simulink model "GFo_29bus"  (R2020a)
settings: Solver=ode1  StartTime=0.0  StopTime=4.5  FixedStep=Time_Step  RelTol=1e-3  EnableMultiTasking=on
PreLoadFcn:
  | Init_29bus;
InitFcn:
  | Init_29bus;
undefined symbols (not defined in the file): D1, D11, Delta, Time_Step, VSC01_Delta_P_Time_Step, VSC01_Delta_P_Value
libraries: powerlib x175, GFo_Lib x1
(part 1 of 5)
Description:
  | Copyright 2008-2017 The MathWorks, Inc.
settings Model: Creator=MathWorks  LastModifiedBy=Frederic_Colas
settings DataIOCC: SaveFormat=StructureWithTime  SignalLoggingSaveFormat=ModelDataLogs  SaveOutput=off  SignalLogging=off  DSMLogging=off  SaveTime=off  ReturnWorkspaceOutputs=off
settings OptimizationCC: ExpressionDepthLimit=2147483647  LifeSpan=inf
settings DebuggingCC: UnderspecifiedInitializationDetection=Classic  MergeDetectMultiDrivingBlocksExec=none  SolverPrmCheckMsg=warning  FcnCallInpInsideContextMsg=warning  UnconnectedInputMsg=none  UnconnectedOutputMsg=none  UnconnectedLineMsg=none  StateNameClashWarn=warning  SFUnexpectedBacktrackingDiag=warning  SFNoUnconditionalDefaultTransitionDiag=warning  SFExecutionAtInitializationDiag=none  ArithmeticOperatorsInVariantConditions=warning
settings HardwareCC: ProdBitPerPointer=32  ProdBitPerSizeT=32  ProdBitPerPtrDiffT=32  ProdLargestAtomicFloat=None  ProdIntDivRoundTo=Undefined  ProdEndianess=Unspecified  ProdWordSize=32  ProdHWDeviceType=32-bit Generic
settings ModelReferenceCC: PropagateSignalLabelsOutOfModel=off
settings SFSimCC: SimUseLocalCustomCode=off  CustomCodeUndefinedFunction=UseInterfaceOnly
settings RTWCC: RTWUseLocalCustomCode=off
settings CodeAppCC: StateflowObjectComments=on
settings GRTTargetCC: TargetLangStandard=C89/C90 (ANSI)  CombineOutputUpdateFcns=off  GRTInterface=on
settings ConfigComp: CovMetricSettings=dw  CovSaveCumulativeToWorkspaceVar=on  CovSaveSingleToWorkspaceVar=on  CovExternalEMLEnable=off  CovSFcnEnable=off
settings SimscapeCC: SimscapeNormalizeSystem=off

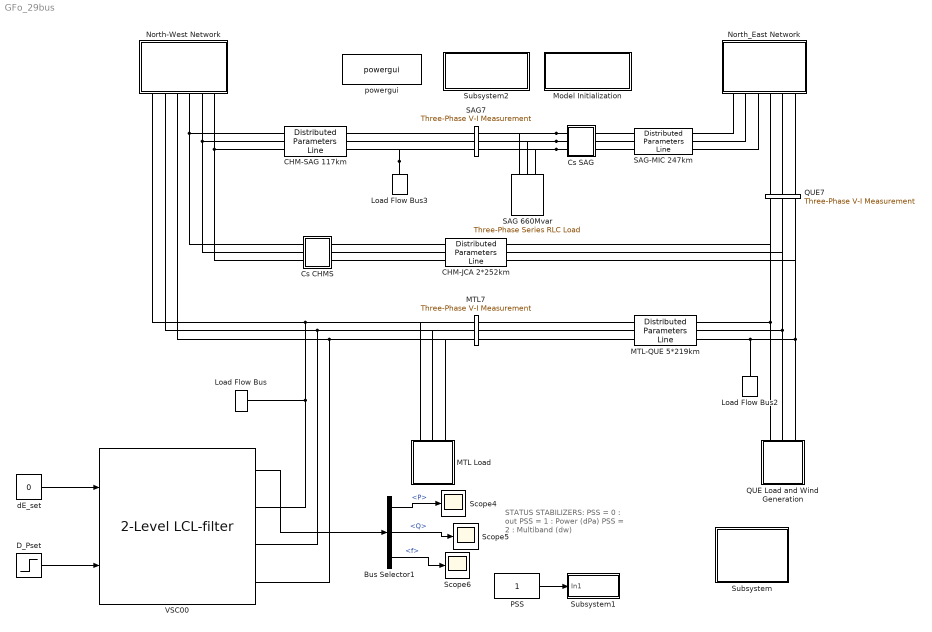
== system GFo_29bus ==
  note: STATUS STABILIZERS:
      | PSS = 0 :  out
      | PSS = 1 :  Power (dPa)
      | PSS = 2 :  Multiband (dw)
  Bus Selector1 : BusSelector  OutputSignals=P,Q,f
  CHM-JCA 2*252km : powerlib/Elements/Distributed Parameters Line  Phases=3  Length=252  Frequency=60  Resistance="[0.01273  0.3864]/2"  Inductance="[0.9337e-3  4.1264e-3]/2"  Capacitance=[12.74e-9 7.751e-9]*2  x1=[-0.00144 1.06587715150696e-07 0 0;-0.0014 1.06951259001269e-07 0 0;-0.00136 1.07290483057854e-07 0 0;-0.00132 1.07605310183825e-07 0 0;-0.00128 1.07895668790209e-07 0 0;-0.00124 1.08161492851963e-07 0 0;-0.0012 1.08402721922987e-07 0 0;-0.00116 1.08619301149872e-07 0 0;-0.00112 1.08811181284367e-07 0 0;-0.00108 1.08978318694587e-07 0 0;-0.00104 1.09120675374924e-07 0 0;-0.001 1.09238218954698e-07 0 0;-0.00096 1.09330922705511e-07 0 0;-0.00092 1.09398765547331e-07 0 0;-0.00088 1.0944173205328e-07 236947.551929989 -735006.025980386;-0.00084 1.09459812453146e-07 248003.849356371 -731349.489712214;-0.0008 1.09453002635601e-07 259003.752846105 -727526.650876972;-0.00076 1.09421304149139e-07 269944.761115994 -723538.378755243;-0.00072 1.09364724201723e-07 280824.38627511 -719385.580245714;-0.00068 1.09283275659145e-07 291640.154390513 -715069.199658954;-0.00064 1.09176977042101e-07 302389.606049806 -710590.218502686;-0.0006 1.09045852521979e-07 313070.296920379 -705949.655258599;-0.00056 1.08889931915365e-07 323679.798305237 -701148.565150758;-0.00052 1.08709250677261e-07 334215.697695255 -696188.039905648;-0.00048 1.08503849893021e-07 344675.599317771 -691069.207503934;-0.00044 1.08273776269012e-07 355057.124681358 -685793.231923961;-0.0004 1.08019082121994e-07 365357.913116674 -680361.312877077;-0.00036 1.07739825367218e-07 375575.62231326 -674774.685534831;-0.00032 1.07436069505262e-07 385707.928852159 -669034.620248103;-0.00028 1.07107883607589e-07 395752.52873424 -663142.42225824;-0.00024 1.06755342300844e-07 405707.137904111 -657099.431400252;-0.0002 1.06378525749878e-07 415569.492769492 -650907.021798148;-0.00016 1.05977519639526e-07 425337.350715936 -644566.60155247;-0.00012 1.05552415155119e-07 435008.49061678 -638079.612420104;-8e-05 1.05103308961751e-07 444580.713338212 -631447.529486439;-4e-05 1.04630303182297e-07 454051.842239331 -624671.860829939]  x2=[-0.00144 7.1019300205437e-08 0 0;-0.0014 7.11442792046729e-08 0 0;-0.00136 7.12530806083399e-08 0 0;-0.00132 7.13456796759369e-08 0 0;-0.00128 7.14220553512345e-08 0 0;-0.00124 7.14821902670629e-08 0 0;-0.0012 7.15260707492606e-08 0 0;-0.00116 7.15536868197846e-08 0 0;-0.00112 7.15650321989784e-08 0 0;-0.00108 7.15601043070008e-08 0 0;-0.00104 7.15389042644118e-08 0 0;-0.001 7.15014368919183e-08 0 0;-0.00096 7.14477107092777e-08 0 0;-0.00092 7.13777379333606e-08 0 0;-0.00088 7.12915344753729e-08 28167.854478783 -750122.429836815;-0.00084 7.11891199372375e-08 39475.8227938335 -749612.37045183;-0.0008 7.10705176071372e-08 50774.8146472057 -748931.855678186;-0.00076 7.09357544542191e-08 62062.2607455905 -748081.040259074;-0.00072 7.0784861122462e-08 73335.5944210838 -747060.117662583;-0.00068 7.06178719237082e-08 84592.2522148251 -745869.320037708;-0.00064 7.04348248298616e-08 95829.6744599052 -744508.91816156;-0.0006 7.02357614642528e-08 107045.305863413 -742979.221377793;-0.00056 7.00207270921744e-08 118236.596087487 -741280.577526264;-0.00052 6.97897706105883e-08 129401.00032924 -739413.372863938;-0.00048 6.95429445370066e-08 140535.979899424 -737378.031977051;-0.00044 6.92803049975501e-08 151639.00279971 -735175.017684571;-0.0004 6.90019117141851e-08 162707.544298438 -732804.830932948;-0.00036 6.87078279911433e-08 173739.087504723 -730268.010682211;-0.00032 6.83981207005275e-08 184731.123940772 -727565.133783408;-0.00028 6.80728602671046e-08 195681.15411229 -724696.814847437;-0.00024 6.77321206522923e-08 206586.688076845 -721663.706105289;-0.0002 6.73759793373407e-08 217445.246010059 -718466.497259735;-0.00016 6.70045173057134e-08 228254.358769498 -715105.915328495;-0.00012 6.66178190246732e-08 239011.568456135 -711582.724478921;-8e-05 6.62159724260743e-08 249714.428973253 -707897.725854228;-4e-05 6.5799068886368e-08 260360.506582668 -704051.757391326]  x3=[-0.00144 2.8189905940601e-10 0 0;-0.0014 2.81135422203296e-10 0 0;-0.00136 2.80307857229982e-10 0 0;-0.00132 2.79416552667206e-10 0 0;-0.00128 2.78461711189939e-10 0 0;-0.00124 2.77443549920899e-10 0 0;-0.0012 2.76362300381179e-10 0 0;-0.00116 2.75218208437598e-10 0 0;-0.00112 2.740115342468e-10 0 0;-0.00108 2.72742552196089e-10 0 0;-0.00104 2.7141155084104e-10 0 0;-0.001 2.70018832839883e-10 0 0;-0.00096 2.68564714884681e-10 0 0;-0.00092 2.67049527629319e-10 0 0;-0.00088 2.6547361561431e-10 329.831041711369 -923.135468483982;-0.00084 2.63837337188458e-10 343.713540361162 -918.056958478673;-0.0008 2.62141064427365e-10 357.517881515936 -912.769690237991;-0.00076 2.6038518304883e-10 371.240926187556 -907.27486604114;-0.00072 2.58570092325136e-10 384.879553874007 -901.573735363756;-0.00068 2.56696204992261e-10 398.430663268966 -895.667594593792;-0.00064 2.54763947156024e-10 411.891172967018 -889.557786736725;-0.0006 2.52773758195194e-10 425.258022164335 -883.245701110174;-0.00056 2.50726090661579e-10 438.528171354681 -876.732773027977;-0.00052 2.48621410177118e-10 451.698603020568 -870.020483473815;-0.00048 2.46460195328001e-10 464.766322319409 -863.110358764447;-0.00044 2.4424293755585e-10 477.72835776453 -856.003970202644;-0.0004 2.41970141045959e-10 490.581761900849 -848.702933719881;-0.00036 2.39642322612656e-10 503.323611975108 -841.208909508892;-0.00032 2.37260011581779e-10 515.951010600483 -833.523601646157;-0.00028 2.34823749670311e-10 528.461086415419 -825.648757704409;-0.00024 2.32334090863202e-10 540.850994736558 -817.586168355251;-0.0002 2.29791601287394e-10 553.117918205594 -809.337666961972;-0.00016 2.27196859083092e-10 565.259067429917 -800.905129162656;-0.00012 2.24550454272297e-10 577.271681616892 -792.290472443681;-8e-05 2.21852988624641e-10 589.153029201647 -783.495655703694;-4e-05 2.1910507552055e-10 600.9004084682 -774.522678808179]  x4=[-0.00144 1.33638805948334e-10 0 0;-0.0014 1.37510109756271e-10 0 0;-0.00136 1.41350144951085e-10 0 0;-0.00132 1.4515803834189e-10 0 0;-0.00128 1.48932924046565e-10 0 0;-0.00124 1.52673943688654e-10 0 0;-0.0012 1.56380246592553e-10 0 0;-0.00116 1.60050989976943e-10 0 0;-0.00112 1.63685339146433e-10 0 0;-0.00108 1.67282467681363e-10 0 0;-0.00104 1.70841557625725e-10 0 0;-0.001 1.74361799673157e-10 0 0;-0.00096 1.77842393350976e-10 0 0;-0.00092 1.81282547202195e-10 0 0;-0.00088 1.84681478965494e-10 -191.737879033871 -10272.5482528801;-0.00084 1.88038415753101e-10 -36.8152546198599 -10274.271133571;-0.0008 1.91352594226541e-10 118.11574126557 -10273.6577336076;-0.00076 1.94623260770207e-10 273.019878650024 -10270.7081924719;-0.00072 1.97849671662735e-10 427.861933668495 -10265.423180864;-0.00068 2.01031093246108e-10 582.606696572975 -10257.80390055;-0.00064 2.04166802092497e-10 737.218979738841 -10247.8520840885;-0.0006 2.07256085168748e-10 891.663625666219 -10235.5699944369;-0.00056 2.10298239998533e-10 1045.9055149745 -10220.9604244363;-0.00052 2.13292574822077e-10 1199.90957438818 -10204.026696177;-0.00048 2.16238408753463e-10 1353.64078471223 -10184.7726602428;-0.00044 2.19135071935459e-10 1507.06418879513 -10163.2026948353;-0.0004 2.21981905691838e-10 1660.14489947787 -10139.3217047788;-0.00036 2.24778262677152e-10 1812.84810752694 -10113.1351204044;-0.00032 2.27523507023939e-10 1965.1390895497 -10084.6488963156;-0.00028 2.30217014487308e-10 2116.98321589014 -10053.8695100341;-0.00024 2.3285817258689e-10 2268.34595850337 -10020.8039605269;-0.0002 2.35446380746108e-10 2419.19289880701 -9985.45976661477;-0.00016 2.37981050428748e-10 2569.4897355077 -9947.84496526266;-0.00012 2.40461605272782e-10 2719.20229240087 -9907.96810975201;-8e-05 2.42887481221429e-10 2868.29652614215 -9865.83826773589;-4e-05 2.45258126651419e-10 3016.73853398852 -9821.46501917704]  x5=0.00142516474882927  V1=ones(3,3)  V2=ones(3,3)  I1=ones(3,3)  I2=ones(3,3)  nHarmo=1  Measurements=None  Decoupling=off  VsMag0=0  VrMag0=0  VsAngle0=0  VrAngle0=0  IsMag0=0  IrMag0=0  IsAngle0=0  IrAngle0=0
      settings: AttributesFormatString=\n
  CHM-SAG 117km : powerlib/Elements/Distributed Parameters Line  Phases=3  Length=117  Frequency=60  Resistance="[0.01273  0.3864]"  Inductance="[0.9337e-3  4.1264e-3]"  Capacitance=[12.74e-9 7.751e-9]  x1=[-0.00068 1.07436413044344e-07 0 0;-0.00064 1.07336181458683e-07 0 0;-0.0006 1.07211542550985e-07 0 0;-0.00056 1.07062524663065e-07 0 0;-0.00052 1.06889161680303e-07 0 0;-0.00048 1.06691493023949e-07 0 0;-0.00044 1.06469563642149e-07 285915.250875085 -721016.735544479;-0.0004 1.06223423999732e-07 296755.036612825 -716623.402961044;-0.00036 1.05953130066728e-07 307527.342814346 -712067.116395673;-0.00032 1.05658743305649e-07 318229.719950114 -707348.911908639;-0.00028 1.05340330657504e-07 328859.734391862 -702469.862378953;-0.00024 1.04997964526583e-07 339414.968965975 -697431.077260406;-0.0002 1.04631722763993e-07 349893.023503134 -692233.702329278;-0.00016 1.04241688649953e-07 360291.515384098 -686878.91942381;-0.00012 1.03827950874855e-07 370608.080081486 -681367.946175457;-8e-05 1.03390603519102e-07 380840.371697451 -675702.03573201;-4e-05 1.02929746031712e-07 390986.063497119 -669882.476472644]  x2=[-0.00068 7.37125407254179e-08 0 0;-0.00064 7.3600352625818e-08 0 0;-0.0006 7.34714284407333e-08 0 0;-0.00056 7.33257974864118e-08 0 0;-0.00052 7.31634928780767e-08 0 0;-0.00048 7.29845515223962e-08 0 0;-0.00044 7.27890141090914e-08 332776.301409299 -689011.544372579;-0.0004 7.2576925101684e-08 343128.151600145 -683915.224594401;-0.00036 7.23483327273852e-08 353401.977408328 -678663.388391983;-0.00032 7.21032889661296e-08 363595.442654457 -673257.22998759;-0.00028 7.18418495387554e-08 373706.22943244 -667697.978695019;-0.00024 7.15640738943339e-08 383732.038636556 -661986.898640076;-0.0002 7.1270025196651e-08 393670.590484249 -656125.288473114;-0.00016 7.0959770309845e-08 403519.625034538 -650114.481073737;-0.00012 7.06333797832015e-08 413276.902701898 -643955.843247712;-8e-05 7.02909278351116e-08 422940.204765532 -637650.775416171;-4e-05 6.99324923361951e-08 432507.333873884 -631200.711297167]  x3=[-0.00068 1.02796560750471e-10 0 0;-0.00064 1.00332195956181e-10 0 0;-0.0006 9.7845016485759e-11 0 0;-0.00056 9.53355879023672e-11 0 0;-0.00052 9.28044808284255e-11 0 0;-0.00048 9.02522708158551e-11 0 0;-0.00044 8.76795382152037e-11 1667.28750300207 -3842.30394709124;-0.0004 8.50868680436783e-11 1725.03630670002 -3816.72583715204;-0.00036 8.24748498521176e-11 1782.3928520179 -3790.27983667152;-0.00032 7.98440775909334e-11 1839.34409657194 -3762.97195924212;-0.00028 7.7195149475051e-11 1895.87709014024 -3734.80841443967;-0.00024 7.45286678478806e-11 1951.9789776076 -3705.7956064114;-0.0002 7.18452390443494e-11 2007.6370018886 -3675.94013241965;-0.00016 6.91454732530265e-11 2062.83850682849 -3645.24878134175;-0.00012 6.64299843773711e-11 2117.57094008109 -3613.72853212625;-8e-05 6.3699389896136e-11 2171.82185596306 -3581.38655220602;-4e-05 6.09543107229587e-11 2225.57891828399 -3548.23019586838]  x4=[-0.00068 1.34957667935224e-10 0 0;-0.00064 1.37600660085736e-10 0 0;-0.0006 1.40212363032762e-10 0 0;-0.00056 1.42792182897574e-10 0 0;-0.00052 1.45339533051383e-10 0 0;-0.00048 1.47853834248731e-10 0 0;-0.00044 1.50334514759208e-10 212.800113433279 -1518.35731016245;-0.0004 1.52781010497458e-10 235.671559776652 -1514.97578249147;-0.00036 1.55192765151448e-10 258.489416439676 -1511.24976239214;-0.00032 1.57569230308969e-10 281.24849483852 -1507.18009712931;-0.00028 1.59909865582336e-10 303.943619755021 -1502.76771210976;-0.00024 1.62214138731274e-10 326.569630513488 -1498.01361067179;-0.0002 1.64481525783939e-10 349.121382154193 -1492.91887385707;-0.00016 1.6671151115607e-10 371.59374660329 -1487.48466016482;-0.00012 1.68903587768222e-10 393.981613838898 -1481.71220528837;-8e-05 1.71057257161078e-10 416.279893053071 -1475.60282183419;-4e-05 1.73172029608791e-10 438.48351380941 -1469.15789902337]  x5=0.000661683633385019  V1=ones(3,3)  V2=ones(3,3)  I1=ones(3,3)  I2=ones(3,3)  nHarmo=1  Measurements=None  Decoupling=off  VsMag0=0  VrMag0=0  VsAngle0=0  VrAngle0=0  IsMag0=0  IrMag0=0  IsAngle0=0  IrAngle0=0
      settings: AttributesFormatString=\n
  Cs CHMS : Subsystem  mask{Xc=33/2}
      mask prompts: Xc "Condensator Reactance at  60Hz  (ohm):"
      mask help: Series Compensation
      mask init:
      | Cs=1/Xc/(2*pi*60);
      mask Display: disp('Cs')
  Cs SAG : Subsystem  mask{Xc=22}
      mask prompts: Xc "Condensator Reactance at  60Hz  (ohm):"
      mask help: Series Compensation
      mask init:
      | Cs=1/Xc/(2*pi*60);
      mask Display: disp('Cs')
  D_Pset : Step  Time=VSC01_Delta_P_Time_Step  After=VSC01_Delta_P_Value  SampleTime=0
  Load Flow Bus : powerlib/Measurements/Load Flow Bus  LConnTagsString=a  Phases=single  Connectors=on one side  ID=BUS_1  Vbase=VSC01_Un2  Vref=1  Vangle=0  VLF=1  VLFb=1  VLFc=1  angleLF=-17.01  angleLFb=0  angleLFc=0
  Load Flow Bus2 : powerlib/Measurements/Load Flow Bus  LConnTagsString=a  Phases=single  Connectors=on one side  ID=QUE7  Vbase=735e3  Vref=1  Vangle=0  VLF=1.021  VLFb=1  VLFc=1  angleLF=-8.842  angleLFb=0  angleLFc=0
      settings: AttributesFormatString=%<ID>\n%<Vbase>V\n%<VLF>pu\n%<angleLF>deg.
  Load Flow Bus3 : powerlib/Measurements/Load Flow Bus  LConnTagsString=a  Phases=single  Connectors=on one side  ID=SAG7  Vbase=735e3  Vref=1  Vangle=0  VLF=1.041  VLFb=1  VLFc=1  angleLF=5.283  angleLFb=0  angleLFc=0
      settings: AttributesFormatString=%<ID>\n%<Vbase>V\n%<VLF>pu\n%<angleLF>deg.
  MTL Load : Subsystem
  MTL-QUE 5*219km : powerlib/Elements/Distributed Parameters Line  Phases=3  Length=219  Frequency=60  Resistance="[0.01273  0.3864]/5"  Inductance="[0.9337e-3  4.1264e-3]/5"  Capacitance=[12.74e-9 7.751e-9]*5  x1=[-0.00124 4.26311042674069e-07 -175262.845803811 -713799.758659779;-0.0012 4.27570122954984e-07 -164479.46915951 -716361.379291687;-0.00116 4.28731977477146e-07 -153658.691302334 -718760.10552358;-0.00112 4.29796342044858e-07 -142802.972783851 -720995.391905801;-0.00108 4.30762974630794e-07 -131914.782100838 -723066.730153502;-0.00104 4.3163165543104e-07 -120996.595133959 -724973.649262228;-0.001 4.32402186915075e-07 -110050.894584778 -726715.715615018;-0.00096 4.33074393870683e-07 -99080.1694112061 -728292.533081006;-0.00092 4.33648123443799e-07 -88086.9142615412 -729703.7431055;-0.00088 4.34123245173266e-07 -77073.6289072024 -730949.024791508;-0.00084 4.344996510205e-07 -66042.8176743049 -732028.094972715;-0.0008 4.34777255394058e-07 -54996.9888741972 -732940.708277866;-0.00076 4.34955995169098e-07 -43938.6542330933 -733686.657186566;-0.00072 4.35035829701737e-07 -32870.3283209276 -734265.772076466;-0.00068 4.35016740838292e-07 -21794.5279795634 -734677.921261835;-0.00064 4.34898732919405e-07 -10713.7717504847 -734923.011023501;-0.0006 4.34681832779058e-07 369.420697898489 -735000.985630166;-0.00056 4.34366089738474e-07 11452.5291432007 -734911.827351078;-0.00052 4.33951575594898e-07 22533.0333821382 -734655.55646006;-0.00048 4.3343838460527e-07 33608.4138036012 -734232.231230902;-0.00044 4.32826633464796e-07 44676.1519615918 -733641.947924112;-0.0004 4.3211646128041e-07 55733.7311478971 -732884.840765022;-0.00036 4.31308029539143e-07 66778.6369643666 -731961.081913272;-0.00032 4.304015220714e-07 77808.3578946649 -730870.881423659;-0.00028 4.29397145009163e-07 88820.3858753686 -729614.487198372;-0.00024 4.28295126739114e-07 99812.2168662786 -728192.184930623;-0.0002 4.27095717850705e-07 110781.351419817 -726604.298039683;-0.00016 4.25799191079173e-07 121725.29524938 -724851.187597338;-0.00012 4.24405841243526e-07 132641.559796518 -722933.252245783;-8e-05 4.22915985179499e-07 143527.662796811 -720850.928106978;-4e-05 4.21329961667516e-07 154381.128844313 -718604.688683476]  x2=[-0.00124 7.14821902670629e-08 -73583.3206395336 -747036.138164079;-0.0012 7.15260707492606e-08 -62310.3261190301 -748060.740679136;-0.00116 7.15536868197846e-08 -51023.1627677086 -748915.240632763;-0.00112 7.15650321989784e-08 -39724.3971891787 -749599.443719041;-0.00108 7.15601043070008e-08 -28416.5986252966 -750113.194356087;-0.00104 7.15389042644118e-08 -17102.3383719414 -750456.375721437;-0.001 7.15014368919183e-08 -5784.18919432479 -750628.909778608;-0.00096 7.14477107092777e-08 5535.27525803398 -750630.757294844;-0.00092 7.13777379333606e-08 16853.4810365332 -750461.917850035;-0.00088 7.12915344753729e-08 28167.854478783 -750122.429836814;-0.00084 7.11891199372375e-08 39475.8227938335 -749612.37045183;-0.0008 7.10705176071372e-08 50774.8146472057 -748931.855678186;-0.00076 7.09357544542191e-08 62062.2607455905 -748081.040259074;-0.00072 7.0784861122462e-08 73335.5944210839 -747060.117662583;-0.00068 7.06178719237082e-08 84592.2522148251 -745869.320037708;-0.00064 7.04348248298616e-08 95829.6744599052 -744508.91816156;-0.0006 7.02357614642528e-08 107045.305863413 -742979.221377793;-0.00056 7.00207270921744e-08 118236.596087487 -741280.577526264;-0.00052 6.97897706105883e-08 129401.00032924 -739413.372863938;-0.00048 6.95429445370066e-08 140535.979899424 -737378.031977051;-0.00044 6.92803049975501e-08 151639.00279971 -735175.017684571;-0.0004 6.90019117141851e-08 162707.544298438 -732804.830932948;-0.00036 6.87078279911433e-08 173739.087504723 -730268.010682211;-0.00032 6.83981207005275e-08 184731.123940772 -727565.133783408;-0.00028 6.80728602671046e-08 195681.15411229 -724696.814847437;-0.00024 6.77321206522923e-08 206586.688076845 -721663.706105289;-0.0002 6.73759793373407e-08 217445.246010059 -718466.497259735;-0.00016 6.70045173057134e-08 228254.358769498 -715105.915328495;-0.00012 6.66178190246732e-08 239011.568456135 -711582.724478921;-8e-05 6.62159724260743e-08 249714.428973253 -707897.725854228;-4e-05 6.5799068886368e-08 260360.506582668 -704051.757391326]  x3=[-0.00124 2.53310769052049e-09 -7027.03988726015 -19339.1228874494;-0.0012 2.47415162952708e-09 -6734.62515237613 -19442.8845645253;-0.00116 2.41463296778928e-09 -6440.67902180939 -19542.2250973194;-0.00112 2.35456523933752e-09 -6145.26833637514 -19637.1218966514;-0.00108 2.29396210305524e-09 -5848.46026991574 -19727.5533838074;-0.00104 2.23283733957301e-09 -5550.32231402593 -19813.4989954472;-0.001 2.17120484813493e-09 -5250.92226270586 -19894.9391882797;-0.00096 2.10907864343806e-09 -4950.32819694527 -19971.8554435074;-0.00092 2.04647285244559e-09 -4648.6084692425 -20044.2302710372;-0.00088 1.9834017111745e-09 -4345.83168806173 -20112.0472134575;-0.00084 1.91987956145842e-09 -4042.06670223194 -20175.2908497803;-0.0008 1.8559208476864e-09 -3737.38258529137 -20233.9467989482;-0.00076 1.7915401135184e-09 -3431.84861978071 -20288.0017231041;-0.00072 1.72675199857817e-09 -3125.53428148892 -20337.4433306245;-0.00068 1.66157123512433e-09 -2818.50922365498 -20382.2603789142;-0.00064 1.59601264470041e-09 -2510.84326112936 -20422.4426769628;-0.0006 1.53009113476451e-09 -2202.60635449876 -20457.9810876623;-0.00056 1.46382169529951e-09 -1893.86859417761 -20488.8675298845;-0.00052 1.39721939540446e-09 -1584.70018447017 -20515.094980319;-0.00048 1.330299379868e-09 -1275.17142760666 -20536.6574750696;-0.00044 1.26307686572457e-09 -965.352707757116 -20553.5501110109;-0.0004 1.19556713879418e-09 -655.314475026678 -20565.7690469033;-0.00036 1.12778555020657e-09 -345.12722943581 -20573.311504266;-0.00032 1.05974751291045e-09 -34.8615048892187 -20576.1757680094;-0.00028 9.91468498168763e-10 275.412146862951 -20574.3611868244;-0.00024 9.22964032040655e-10 585.623172267978 -20567.8681733314;-0.0002 8.54249691850964e-10 895.701032013831 -20556.6982039854;-0.00016 7.85341102648081e-10 1205.5752170692 -20540.8538187413;-0.00012 7.1625393365095e-10 1515.17526471665 -20520.3386204756;-8e-05 6.47003894686017e-10 1824.43077457521 -20495.1572741674;-4e-05 5.77606732614956e-10 2133.27142460885 -20465.3155058379]  x4=[-0.00124 4.49447007897503e-10 -1381.07232419638 -6777.19407552042;-0.0012 5.27984712516739e-10 -1278.72088950854 -6797.2485342467;-0.00116 6.06402357965495e-10 -1176.07868471766 -6815.75735727326;-0.00112 6.84682112747441e-10 -1073.16904977593 -6832.71633585337;-0.00108 7.62806176721395e-10 -970.015385446906 -6848.12161366153;-0.00104 8.40756785148923e-10 -866.641147984285 -6861.96968767044;-0.001 9.18516212733886e-10 -763.069843798208 -6874.25740894748;-0.00096 9.9606677765302e-10 -659.325024110085 -6884.9819833708;-0.00092 1.07339084557663e-09 -555.430279597257 -6894.14097226465;-0.00088 1.15047083367848e-09 -451.409235028674 -6901.73229295395;-0.00084 1.227289214634e-09 -347.285543892834 -6907.75421923783;-0.0008 1.30382852060579e-09 -243.082883019175 -6912.2053817822;-0.00076 1.38007134721574e-09 -138.824947194175 -6915.08476843107;-0.00072 1.45600035750256e-09 -34.5354437733588 -6916.39172443675;-0.00068 1.5315982858641e-09 69.7619127095507 -6916.12595260871;-0.00064 1.60684794198337e-09 174.043405935111 -6914.28751338119;-0.0006 1.6817322147375e-09 278.285323191048 -6910.87682479939;-0.00056 1.75623407608865e-09 382.463960764322 -6905.8946624245;-0.00052 1.830336584956e-09 486.555629331147 -6899.34215915727;-0.00048 1.90402289106809e-09 590.536659343739 -6891.22080498044;-0.00044 1.97727623879435e-09 694.383406412568 -6881.53244661992;-0.0004 2.0500799709552e-09 798.072256682885 -6870.27928712485;-0.00036 2.1224175326098e-09 901.579632204316 -6857.46388536664;-0.00032 2.19427247482043e-09 1004.88199629227 -6843.08915545716;-0.00028 2.26562845839289e-09 1107.95585888001 -6827.15836608601;-0.00024 2.33646925759185e-09 1210.77778186004 -6809.67513977732;-0.0002 2.40677876383049e-09 1313.32438441378 -6790.64345206598;-0.00016 2.47654098933342e-09 1415.57234832813 -6770.06763059366;-0.00012 2.54574007077215e-09 1517.49842329784 -6747.95235412472;-8e-05 2.61436027287231e-09 1619.07943221245 -6724.30265148231;-4e-05 2.6823859919917e-09 1720.29227642652 -6699.12390040487]  x5=0.00123853603172068  V1=ones(3,3)  V2=ones(3,3)  I1=ones(3,3)  I2=ones(3,3)  nHarmo=1  Measurements=None  Decoupling=off  VsMag0=0  VrMag0=0  VsAngle0=0  VrAngle0=0  IsMag0=0  IrMag0=0  IsAngle0=0  IrAngle0=0
      settings: AttributesFormatString=\n
  MTL7 : powerlib/Measurements/Three-Phase V-I Measurement  VoltageMeasurement=phase-to-ground  SetLabelV=on  LabelV=Vabc_MTL7  Vpu=on  VpuLL=off  CurrentMeasurement=no  SetLabelI=off  LabelI=A1  Ipu=off  Pbase=100e6  Vbase=735e3  OutputType=Magnitude  PhasorSimulation=off  PSBequivalent=0
  Model Initialization : Subsystem  mask(Model Functions){InitFcnX=Init_29bus;, prel=on, posl=off, inif=on, strf=off}
      mask prompts: InitFcnX "Initialisation"; prel "Preload Function"; posl "PostLoad Function"; inif "InitFcn"; strf "StartFcn"
      mask init:
      | currentBlock = gcb;
      | root = bdroot(currentBlock);
      | 
      | if ~strcmp(get_param(root,'BlockDiagramType'),'library')
      |     if prel==1
      |         set_param(root, 'PreLoadFcn', InitFcnX);
      |     else
      |         set_param(root, 'PreLoadFcn', '');
      |     end
      |     if inif==1
      |         set_param(root, 'InitFcn', InitFcnX);
      |     else
      |         set_param(root, 'InitFcn', '');
      |     end
      |     if strf==1
      |         set_param(root, 'StartFcn', InitFcnX);
      |     else
      |         set_param(root, 'StartFcn', '');
      |     end
      |     if posl==1
      |         set_param(root, 'PostLoadFcn', InitFcnX);
      |     else
      |         set_param(root, 'PostLoadFcn', '');
      |     end
      | end
      | 
      | pos = get_param(currentBlock, 'Position');
      | width = pos(3) - pos(1); height = pos(4) - pos(2);
      | txt = [ upper(root) '\n' '- InitFcn. . . . . '  get_param(root, 'InitFcn') ];
      settings: CopyFcn=set_param(gcb,'LinkStatus','none')
      mask Display:
      | %text(5, height*0.5, txt, 'horizontalAlignment', 'left', 'verticalAlignment', 'middle') ;
      | color('blue'),disp('Initialization Function\nParameters')
  North-West Network : Subsystem
  North_East Network : Subsystem
  PSS : Constant
  QUE Load and Wind Generation : Subsystem
  QUE7 : powerlib/Measurements/Three-Phase V-I Measurement  VoltageMeasurement=no  SetLabelV=on  LabelV=Vabc_QUE7  Vpu=on  VpuLL=off  CurrentMeasurement=no  SetLabelI=off  LabelI=A1  Ipu=off  Pbase=100e6  Vbase=735e3  OutputType=Magnitude  PhasorSimulation=off  PSBequivalent=0
  SAG 660Mvar : powerlib/Elements/Three-Phase Series RLC Load  LConnTagsString=A|B|C  Configuration=Y (grounded)  NominalVoltage=735e3  Vabc=[1e3 1e3 1e3]  Vabcp=[1e3 1e3 1e3]  NominalFrequency=60  UnbalancedPower=off  ActivePower=2200000  InductivePower=660e6  CapacitivePower=0  Pabc=[10e3 9e3 11e3]  QLabc=[100 90 110]  QCabc=[100 90 110]  Pabcp=[10e3 9e3 11e3]  QLabcp=[100 90 110]  QCabcp=[100 90 110]  Measurements=None  LoadType=constant Z
  SAG-MIC 247km : powerlib/Elements/Distributed Parameters Line  Phases=3  Length=247  Frequency=60  Resistance="[0.01273  0.3864]/1"  Inductance="[0.9337e-3  4.1264e-3]/1"  Capacitance=[12.74e-9 7.751e-9]*1  x1=[-0.0014 7.5207848908823e-08 36522.5847826561 -754650.708754004;-0.00136 7.53940710427611e-08 47897.885035945 -754014.151845115;-0.00132 7.55631492151149e-08 59262.2937232307 -753206.138620438;-0.00128 7.5715044978966e-08 70613.2266759799 -752226.852815211;-0.00124 7.58497237945276e-08 81948.1027899254 -751076.517110582;-0.0012 7.59671550369986e-08 93264.344611987 -749755.393082971;-0.00116 7.60673120035269e-08 104559.378926361 -748263.781144587;-0.00112 7.61501719192822e-08 115830.637339649 -746602.020475123;-0.00108 7.62157159426342e-08 127075.556864887 -744770.488944625;-0.00104 7.62639291694371e-08 138291.580504347 -742769.603027567;-0.001 7.62948006364191e-08 149476.157830976 -740599.817708154;-0.00096 7.63083233236747e-08 160626.745568341 -738261.626376854;-0.00092 7.63044941562614e-08 171740.80816895 -735755.560718214;-0.00088 7.62833140048989e-08 182815.818390812 -733082.190589952;-0.00084 7.6244787685771e-08 193849.257872108 -730242.123893382;-0.0008 7.61889239594303e-08 204838.617703848 -727236.006435178;-0.00076 7.61157355288066e-08 215781.399000376 -724064.521780526;-0.00072 7.60252390363178e-08 226675.11346759 -720728.391097689;-0.00068 7.59174550600859e-08 237517.283968765 -717228.372994012;-0.00064 7.57924081092576e-08 248305.445087827 -713565.263343431;-0.0006 7.56501266184311e-08 259037.143689972 -709739.895105491;-0.00056 7.54906429411905e-08 269709.939479482 -705753.138135939;-0.00052 7.53139933427486e-08 280321.405554634 -701605.898988932;-0.00048 7.51202179917008e-08 290869.128959552 -697299.120710885;-0.00044 7.49093609508909e-08 301350.711232893 -692833.782626041;-0.0004 7.46814701673916e-08 311763.768953237 -688210.900113772;-0.00036 7.44365974616017e-08 322105.934281058 -683431.524377694;-0.00032 7.4174798515463e-08 332374.855497146 -678496.742206636;-0.00028 7.38961328597981e-08 342568.197537374 -673407.675727507;-0.00024 7.36006638607739e-08 352683.642523663 -668165.482150137;-0.0002 7.3288458705493e-08 362718.890291057 -662771.353504141;-0.00016 7.29595883867151e-08 372671.658910753 -657226.516367854;-0.00012 7.26141276867148e-08 382539.685208996 -651532.231589426;-8e-05 7.22521551602761e-08 392320.725281705 -645689.794000108;-4e-05 7.187375311683e-08 402012.555004714 -639700.532119827]  x2=[-0.0014 2.56600194395947e-08 154421.7250771 -749560.143875039;-0.00136 2.57201073198396e-08 165706.858589731 -747146.344688975;-0.00132 2.57743466694807e-08 176954.311791714 -744562.650867245;-0.00128 2.58227251549576e-08 188161.527109185 -741809.649919542;-0.00124 2.586523177542e-08 199325.956118026 -738887.967854542;-0.0012 2.5901856865229e-08 210445.060123361 -735798.26903755;-0.00116 2.59325920961549e-08 221516.310736824 -732541.256039432;-0.00112 2.59574304792712e-08 232537.190451501 -729117.669476858;-0.00108 2.5976366366544e-08 243505.193214384 -725528.287843889;-0.00104 2.59893954521156e-08 254417.82499623 -721773.927334952;-0.001 2.59965147732844e-08 265272.604358678 -717855.441659253;-0.00096 2.59977227111782e-08 276067.063018508 -713773.721846643;-0.00092 2.59930189911222e-08 286798.746408909 -709529.696045007;-0.00088 2.59824046827019e-08 297465.214237623 -705124.329309214;-0.00084 2.59658821995195e-08 308064.04104185 -700558.623381669;-0.0008 2.59434552986452e-08 318592.816739776 -695833.616464527;-0.00076 2.59151290797627e-08 329049.147178602 -690950.382983615;-0.00072 2.58809099840101e-08 339430.654678959 -685910.033344115;-0.00068 2.58408057925146e-08 349734.978575568 -680713.713678069;-0.00064 2.57948256246235e-08 359959.775754034 -675362.605583757;-0.0006 2.57429799358304e-08 370102.721183655 -669857.925857014;-0.00056 2.5685280515398e-08 380161.508446108 -664200.926214541;-0.00052 2.56217404836767e-08 390133.850259914 -658392.893009271;-0.00048 2.5552374289122e-08 400017.479000542 -652435.146937869;-0.00044 2.54771977050082e-08 409810.147216049 -646329.042740415;-0.0004 2.53962278258423e-08 419509.628138131 -640075.968892345;-0.00036 2.53094830634765e-08 429113.716188472 -633677.34728873;-0.00032 2.52169831429218e-08 438620.227480271 -627134.632920942;-0.00028 2.51187490978624e-08 448027.00031484 -620449.313545806;-0.00024 2.5014803265873e-08 457331.895673158 -613622.909347297;-0.0002 2.49051692833394e-08 466532.797702262 -606656.972590861;-0.00016 2.47898720800838e-08 475627.614196376 -599553.087270445;-0.00012 2.46689378736959e-08 484614.27707266 -592312.868748309;-8e-05 2.45423941635714e-08 493490.742841473 -584937.963387709;-4e-05 2.44102697246588e-08 502254.993071046 -577430.048178524]  x3=[-0.0014 8.14946303305368e-11 -207.547752866079 -4152.74770849199;-0.00136 8.02445812459464e-11 -144.904646864587 -4155.4050749819;-0.00132 7.89762852355805e-11 -82.2285907960024 -4157.11753819245;-0.00128 7.76900306990145e-11 -19.5338366549794 -4157.88470872427;-0.00124 7.63861101194379e-11 43.1653593120458 -4157.70641212939;-0.0012 7.50648199971458e-11 105.854739848606 -4156.58268895094;-0.00116 7.37264607821178e-11 168.520049930177 -4154.51379471385;-0.00112 7.23713368056979e-11 231.147040005649 -4151.50019986685;-0.00108 7.09997562113922e-11 293.72146923755 -4147.54258967541;-0.00104 6.96120308847999e-11 356.229108740293 -4142.64186406597;-0.001 6.82084763826929e-11 418.655744815698 -4136.79913742125;-0.00096 6.67894118612614e-11 480.987182185065 -4130.01573832693;-0.00092 6.53551600035399e-11 543.20924721706 -4122.29320926945;-0.00088 6.39060469460326e-11 605.307791150674 -4113.63330628532;-0.00084 6.2442402204552e-11 667.268693312533 -4104.0379985618;-0.0008 6.09645585992904e-11 729.077864327813 -4093.50946798913;-0.00076 5.94728521791393e-11 790.721249324045 -4082.05010866436;-0.00072 5.79676221452748e-11 852.18483112707 -4069.66252634698;-0.00068 5.64492107740258e-11 913.454633448425 -4056.34953786639;-0.00064 5.49179633390441e-11 974.516724063432 -4042.11417048135;-0.0006 5.33742280327915e-11 1035.35721797926 -4026.95966119165;-0.00056 5.18183558873639e-11 1095.96228059226 -4010.88945600202;-0.00052 5.025070069467e-11 1156.31813083383 -3993.90720913854;-0.00048 4.86716189259818e-11 1216.41104430411 -3976.01678221768;-0.00044 4.70814696508759e-11 1276.2273563928 -3957.22224336825;-0.0004 4.54806144555847e-11 1335.75346538636 -3937.52786630632;-0.00036 4.38694173607745e-11 1394.97583556094 -3916.93812936338;-0.00032 4.22482447387701e-11 1453.88100026028 -3895.45771446806;-0.00028 4.06174652302455e-11 1512.45556495788 -3873.09150608146;-0.00024 3.89774496603977e-11 1570.68621030288 -3849.8445900865;-0.0002 3.73285709546242e-11 1628.55969514868 -3825.7222526314;-0.00016 3.56712040537236e-11 1686.0628595639 -3800.72997892768;-0.00012 3.40057258286366e-11 1743.18262782484 -3774.87345200285;-8e-05 3.23325149947489e-11 1799.90601138879 -3748.15855140815;-4e-05 3.06519520257752e-11 1856.22011184747 -3720.59135188161]  x4=[-0.0014 3.69661890515573e-11 11.9349515087922 -1468.59968146897;-0.00136 3.90442754177583e-11 34.0788908832543 -1468.25257093725;-0.00132 4.11134834524328e-11 56.2150810118136 -1467.57159243257;-0.00128 4.31733426355177e-11 78.3384883157289 -1466.55690080356;-0.00124 4.52233845727984e-11 100.444082122964 -1465.20872678237;-0.0012 4.72631431024171e-11 122.526835812116 -1463.52737693212;-0.00116 4.92921544008743e-11 144.581727955432 -1461.51323357728;-0.00112 5.13099570884982e-11 166.60374346063 -1459.16675471668;-0.00108 5.33160923343584e-11 188.587874711295 -1456.48847391938;-0.00104 5.53101039606001e-11 210.529122705563 -1453.47900020333;-0.001 5.72915385461752e-11 232.422498192853 -1450.1390178969;-0.00096 5.92599455299461e-11 254.263022808381 -1446.46928648326;-0.00092 6.12148773131395e-11 276.045730205193 -1442.4706404277;-0.00088 6.31558893611266e-11 297.765667183473 -1438.14398898785;-0.00084 6.5082540304506e-11 319.417894816858 -1433.49031600692;-0.0008 6.69943920394682e-11 340.997489575504 -1428.51067969003;-0.00076 6.88910098274156e-11 362.499544445657 -1423.20621236353;-0.00072 7.07719623938191e-11 383.919170045467 -1417.57812021754;-0.00068 7.26368220262856e-11 405.251495736786 -1411.62768303169;-0.00064 7.44851646718166e-11 426.491670732715 -1405.35625388408;-0.0006 7.63165700332339e-11 447.634865200626 -1398.76525884361;-0.00056 7.81306216647517e-11 468.676271360429 -1391.85619664572;-0.00052 7.99269070666728e-11 489.611104577818 -1384.63063835157;-0.00048 8.17050177791871e-11 510.434604452251 -1377.0902269908;-0.00044 8.34645494752526e-11 531.142035899433 -1369.23667718793;-0.0004 8.5205102052535e-11 551.728690228025 -1361.07177477247;-0.00036 8.69262797243882e-11 572.189886210365 -1352.5973763728;-0.00032 8.86276911098523e-11 592.520971146935 -1343.81540899405;-0.00028 9.03089493226508e-11 612.717321924351 -1334.72786957987;-0.00024 9.19696720591644e-11 632.774346066609 -1325.33682455835;-0.0002 9.36094816853645e-11 652.687482779386 -1315.64440937214;-0.00016 9.52280053226831e-11 672.452203987116 -1305.65282799287;-0.00012 9.68248749328027e-11 692.06401536264 -1295.36435241999;-8e-05 9.83997274013448e-11 711.518457349177 -1284.78132216411;-4e-05 9.99522046204388e-11 730.811106174386 -1273.90614371506]  x5=0.00139688767047948  V1=ones(3,3)  V2=ones(3,3)  I1=ones(3,3)  I2=ones(3,3)  nHarmo=1  Measurements=None  Decoupling=off  VsMag0=0  VrMag0=0  VsAngle0=0  VrAngle0=0  IsMag0=0  IrMag0=0  IsAngle0=0  IrAngle0=0
      settings: AttributesFormatString=\n
  SAG7 : powerlib/Measurements/Three-Phase V-I Measurement  VoltageMeasurement=no  SetLabelV=on  LabelV=Vabc_SAG7  Vpu=on  VpuLL=off  CurrentMeasurement=no  SetLabelI=off  LabelI=Iabc_SAG7  Ipu=off  Pbase=100e6  Vbase=735e3  OutputType=Magnitude  PhasorSimulation=off  PSBequivalent=0
  Scope4 : Scope
  Scope5 : Scope
  Scope6 : Scope
  Subsystem : Subsystem
      mask Display: disp('Display\nWaveforms')
  Subsystem1 : Subsystem
      mask Display: disp('PSS_select')
  Subsystem2 : Subsystem
      settings: OpenFcn=LoadFlow_VSC
      mask Display: color('blue'),disp('Update Loadflow')
  VSC00 : GFo_Lib/2-Level LCL-filter  fn=fb  Sn=VSC01_Sn  Pn=VSC01_Pn  Udcn=VSC01_Udc_n  Time_Step=Time_Step  bridge_type=Average (no switches)  fpwm=4e3  Un1=VSC01_Un1  Un2=VSC01_Un2  Rt_pu=VSC01_Rt_pu  Lt_pu=VSC01_Lt_pu  Rm_pu=500  Lm_pu=500  Lf_pu=VSC01_Lf_pu  Rf_pu=VSC01_Rf_pu  Cf_pu=VSC01_Cf_pu  H_DC=40  Tr_PLL=VSC01_Tr_PLL  Val_Freq_Support=on  Val_gamma=on  R_percent=VSC01_R  Rv=VSC01_Rv  W_TVR=VSC01_W_LF  I_Max_VI_pu=1.2  DX_DR=5  Val_Mod_H=off  RLCL_D=0.7  f_damping=200  I_max_pu=1.2  Tr_I_max=10  Advanced=off  gainpopup=With Inertia  f_Inertia_Less=3  zeta_Inertia_Less=1  Tr_Inertia_Less=100  Param_Inertia=PI  H_GFo=5  zeta_GFo=1  LFpopup=PV  P0=0.9  Q0=-0.3128  V0=1  Theta0=-17.0119
      settings: SourceProductName=VSC4SPS
  dE_set : Constant  Value=0
  powergui : powerlib/powergui  Priority=1  SimulationMode=Discrete  SampleTime=Time_Step  frequency=60  Iterations=50  frequencyindice=60  Pbase=5500000000  ErrMax=1e-6  UnitsV=kV  UnitsW=MW  buscounter=0  FunctionMessages=off  echomessages=off  EnableUseOfTLC=off  CurrentSourceSwitches=off  DisableSnubberDevices=off  DisableRonSwitches=off  DisableVfSwitches=off  DisplayEquations=off  AutomaticDiscreteSolvers=off  SolverType=Tustin/Backward Euler (TBE)  Interpol=off  ExternalGateDelay=off  methode=off  Ts=100  x0status=blocks  SPID=off  SwTol=0  HookPort=off  NonlinearTolerance=1e-4  nMaxIteration=100  ContinueOnMaxIteration=off  RestoreLinks=warning  ResistiveCurrentMeasurement=off  Frange=[0:2:500]  Ylog=off  Xlog=on  ShowGrid=off  save=off  variable=ZData  structure=0  ZoomFFT=off  StartTime=0.0  cycles=1  DisplayStyle=1  fundamental=60  FreqAxis=off  MaxFrequency=1000  frequencyindicesteady=1  RmsSteady=1  display=off
  wires:
  PSS/1 -> Subsystem1/1(In1)
  D_Pset/1 -> VSC00/2
  dE_set/1 -> VSC00/1
  Bus Selector1/3 -> Scope6/1  "<f>"
  Bus Selector1/2 -> Scope5/1  "<Q>"
  VSC00/1 -> Bus Selector1/1
  Bus Selector1/1 -> Scope4/1  "<P>"
  connections:
  QUE Load and Wind Generation/LConn3 -- MTL-QUE 5*219km/RConn3 -- Load Flow Bus2/LConn1 -- CHM-JCA 2*252km/RConn3 -- QUE7/LConn3
  MTL7/RConn1 -- MTL-QUE 5*219km/LConn1
  MTL7/RConn2 -- MTL-QUE 5*219km/LConn2
  MTL7/RConn3 -- MTL-QUE 5*219km/LConn3
  QUE Load and Wind Generation/LConn2 -- MTL-QUE 5*219km/RConn2 -- CHM-JCA 2*252km/RConn2 -- QUE7/LConn2
  QUE Load and Wind Generation/LConn1 -- MTL-QUE 5*219km/RConn1 -- CHM-JCA 2*252km/RConn1 -- QUE7/LConn1
  Cs SAG/LConn1 -- SAG7/RConn1 -- SAG 660Mvar/LConn1
  Cs SAG/LConn2 -- SAG7/RConn2 -- SAG 660Mvar/LConn2
  Cs SAG/LConn3 -- SAG7/RConn3 -- SAG 660Mvar/LConn3
  Load Flow Bus3/LConn1 -- CHM-SAG 117km/RConn3 -- SAG7/LConn3
  Cs CHMS/LConn1 -- CHM-SAG 117km/LConn1 -- North-West Network/RConn4
  Cs CHMS/LConn2 -- CHM-SAG 117km/LConn2 -- North-West Network/RConn5
  Cs CHMS/LConn3 -- CHM-SAG 117km/LConn3 -- North-West Network/RConn6
  Cs SAG/RConn1 -- SAG-MIC 247km/LConn1
  Cs SAG/RConn3 -- SAG-MIC 247km/LConn3
  Cs CHMS/RConn3 -- CHM-JCA 2*252km/LConn3
  Cs CHMS/RConn2 -- CHM-JCA 2*252km/LConn2
  Cs CHMS/RConn1 -- CHM-JCA 2*252km/LConn1
  Cs SAG/RConn2 -- SAG-MIC 247km/LConn2
  SAG7/LConn2 -- CHM-SAG 117km/RConn2
  SAG7/LConn1 -- CHM-SAG 117km/RConn1
  SAG-MIC 247km/RConn1 -- North_East Network/LConn1
  SAG-MIC 247km/RConn2 -- North_East Network/LConn2
  SAG-MIC 247km/RConn3 -- North_East Network/LConn3
  QUE7/RConn1 -- North_East Network/LConn4
  QUE7/RConn2 -- North_East Network/LConn5
  QUE7/RConn3 -- North_East Network/LConn6
  MTL7/LConn1 -- MTL Load/LConn1 -- Load Flow Bus/LConn1 -- VSC00/RConn1 -- North-West Network/RConn1
  MTL7/LConn2 -- MTL Load/LConn2 -- VSC00/RConn2 -- North-West Network/RConn2
  MTL7/LConn3 -- MTL Load/LConn3 -- VSC00/RConn3 -- North-West Network/RConn3

== system GFo_29bus/Cs CHMS ==
  note: B
  Ca : powerlib/Elements/Series RLC Branch  LConnTagsString=__new0  RConnTagsString=__new0  BranchType=C  Resistance=1.0  Inductance=1.0  SetiL0=off  InitialCurrent=0  Capacitance=Cs  Setx0=off  InitialVoltage=0  Measurements=None
  Cb : powerlib/Elements/Series RLC Branch  LConnTagsString=__new0  RConnTagsString=__new0  BranchType=C  Resistance=1.0  Inductance=1.0  SetiL0=off  InitialCurrent=0  Capacitance=Cs  Setx0=off  InitialVoltage=0  Measurements=None
  Cc : powerlib/Elements/Series RLC Branch  LConnTagsString=__new0  RConnTagsString=__new0  BranchType=C  Resistance=1.0  Inductance=1.0  SetiL0=off  InitialCurrent=0  Capacitance=Cs  Setx0=off  InitialVoltage=0  Measurements=None
  A : PMIOPort  Side=Left
  B : PMIOPort  Port=2  Side=Left
  C : PMIOPort  Port=3  Side=Left
  "A " : PMIOPort  Port=4  Side=Right
  "B " : PMIOPort  Port=5  Side=Right
  "C " : PMIOPort  Port=6  Side=Right
  connections:
  Cc/RConn1 -- "C "/RConn1
  C/RConn1 -- Cc/LConn1
  Cb/RConn1 -- "B "/RConn1
  B/RConn1 -- Cb/LConn1
  Ca/RConn1 -- "A "/RConn1
  A/RConn1 -- Ca/LConn1

== system GFo_29bus/Cs SAG ==
  note: B
  Ca : powerlib/Elements/Series RLC Branch  LConnTagsString=__new0  RConnTagsString=__new0  BranchType=C  Resistance=1.0  Inductance=1.0  SetiL0=off  InitialCurrent=0  Capacitance=Cs  Setx0=off  InitialVoltage=0  Measurements=None
  Cb : powerlib/Elements/Series RLC Branch  LConnTagsString=__new0  RConnTagsString=__new0  BranchType=C  Resistance=1.0  Inductance=1.0  SetiL0=off  InitialCurrent=0  Capacitance=Cs  Setx0=off  InitialVoltage=0  Measurements=None
  Cc : powerlib/Elements/Series RLC Branch  LConnTagsString=__new0  RConnTagsString=__new0  BranchType=C  Resistance=1.0  Inductance=1.0  SetiL0=off  InitialCurrent=0  Capacitance=Cs  Setx0=off  InitialVoltage=0  Measurements=None
  A : PMIOPort  Side=Left
  B : PMIOPort  Port=2  Side=Left
  C : PMIOPort  Port=3  Side=Left
  "A " : PMIOPort  Port=4  Side=Right
  "B " : PMIOPort  Port=5  Side=Right
  "C " : PMIOPort  Port=6  Side=Right
  connections:
  A/RConn1 -- Ca/LConn1
  Ca/RConn1 -- "A "/RConn1
  B/RConn1 -- Cb/LConn1
  Cb/RConn1 -- "B "/RConn1
  C/RConn1 -- Cc/LConn1
  Cc/RConn1 -- "C "/RConn1

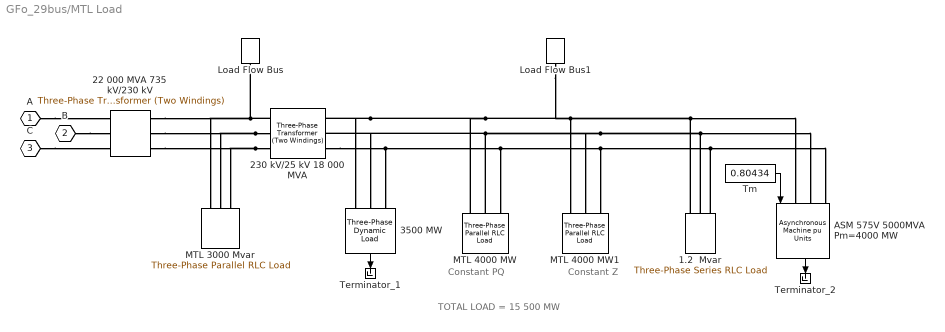
== system GFo_29bus/MTL Load ==
  note: Constant PQ
  note: Constant Z
  note: TOTAL LOAD = 15 500 MW
  1.2  Mvar : powerlib/Elements/Three-Phase Series RLC Load  LConnTagsString=A|B|C  Configuration=Y (grounded)  NominalVoltage=25e3  Vabc=[1e3 1e3 1e3]  Vabcp=[1e3 1e3 1e3]  NominalFrequency=60  UnbalancedPower=off  ActivePower=2000e6/50  InductivePower=0  CapacitivePower=2000e6  Pabc=[10e3 9e3 11e3]  QLabc=[100 90 110]  QCabc=[100 90 110]  Pabcp=[10e3 9e3 11e3]  QLabcp=[100 90 110]  QCabcp=[100 90 110]  Measurements=None  LoadType=constant Z
  22 000 MVA 735 kV/230 kV : powerlib/Elements/Three-Phase Transformer (Two Windings)  Winding1Connection=Yg  Winding2Connection=Delta (D1)  CoreType=Three single-phase transformers  SetSaturation=off  Hysteresis=off  DataFile='basic_model'  SetInitialFlux=off  Measurements=None  UNITS=pu  NominalPower=[ 22000e6 60 ]  Winding1="[ 735e3 0.002  0.12]"  Winding2=[230e3 0.002 0]  Rm=500  Lm=500  L0=0.5  Saturation="[ 0,0  ;  0.005,1.2  ;  1.0,1.4 ]"  InitialFluxes=[ 0.8 , -0.8 , 0.7 ]  BreakLoop=off  DiscreteSolver=Trapezoidal iterative  DataType=off  TransfoNumber=0
  230 kV/25 kV 18 000 MVA : powerlib/Elements/Three-Phase Transformer (Two Windings)  Winding1Connection=Yg  Winding2Connection=Delta (D1)  CoreType=Three single-phase transformers  SetSaturation=off  Hysteresis=off  DataFile='basic_model'  SetInitialFlux=off  Measurements=None  UNITS=pu  NominalPower=[18000e6 60 ]  Winding1="[ 230e3  0.08/30   0.08 ]"  Winding2="[ 25e3  0.08/30  0.08]"  Rm=500  Lm=500  L0=0.5  Saturation="[ 0,0  ;  0.005,1.2  ;  1.0,1.4 ]"  InitialFluxes=[ 0.8 , -0.8 , 0.7 ]  BreakLoop=off  DiscreteSolver=Trapezoidal iterative  DataType=off  TransfoNumber=0
  3500 MW : powerlib/Elements/Three-Phase Dynamic Load  NominalVoltage=[ 25e3 60 ]  ActiveReactivePowers=[3.5e+09 -7.6626e-08]  PositiveSequence=[0.977579 -90.0235]  ExternalControl=off  NpNq="[1.5  2.5]"  TimeConstants="[0  0  0  0]"  MinimumVoltage=0.7  Tfilter=1e-4  LoadFlowParameters=[4,0,0,0,0]
      settings: SourceProductBaseCode=PS
  ASM 575V 5000MVA Pm=4000 MW : powerlib/Machines/Asynchronous Machine pu Units  RotorType=Squirrel-cage  PresetModel=No  MechanicalLoad=Torque Tm  ShowDetailedParameters=on  ReferenceFrame=Rotor  Units=pu  MeasurementBus=off  NominalParameters="[5000e6 25e3  60]"  VoltageRatio=1  Stator=[0.01117 0.04832]  Rotor=[0.006 0.04832]  Cage1=[0.01909 0.0397]  Cage2=[0.01909 0.0397]  Lm=2.424  Mechanical="[1  0   2]"  PolePairs=2  InitialConditions=[0.00539423 0 0.951058 0.951058 0.951058 -118.861 -238.861 1.13934]  SimulateSaturation=off  Saturation="[0.212,0.4201,0.8125,1.0979,1.4799,2.2457,3.2586,4.5763,6.4763 ;   0.5,0.7,0.9,1,1.1,1.2 ,1.3,1.4,1.5]"  LoadFlowParameters=0  TsPowergui=0  TsBlock=-1  IterativeModel=Trapezoidal non iterative  IterativeDiscreteModel=Trapezoidal non iterative  Pmec=4000000000
      settings: SourceProductBaseCode=PS
  Load Flow Bus : powerlib/Measurements/Load Flow Bus  LConnTagsString=a  Phases=single  Connectors=on one side  ID=MTL2  Vbase=230e3  Vref=1  Vangle=0  VLF=0.9954  VLFb=1  VLFc=1  angleLF=-51.92  angleLFb=0  angleLFc=0
      settings: AttributesFormatString=%<ID>\n%<Vbase>V\n%<VLF>pu\n%<angleLF>deg.
  Load Flow Bus1 : powerlib/Measurements/Load Flow Bus  LConnTagsString=a  Phases=single  Connectors=on one side  ID=MTL_25  Vbase=25e3  Vref=1  Vangle=0  VLF=0.9776  VLFb=1  VLFc=1  angleLF=-90.02  angleLFb=0  angleLFc=0
      settings: AttributesFormatString=%<ID>\n%<Vbase>V\n%<VLF>pu\n%<angleLF>deg.
  MTL 3000 Mvar : powerlib/Elements/Three-Phase Parallel RLC Load  LConnTagsString=A|B|C  Configuration=Y (grounded)  NominalVoltage=230e3  Vabc=[1e3 1e3 1e3]  Vabcp=[1e3 1e3 1e3]  NominalFrequency=60  UnbalancedPower=off  ActivePower=0  InductivePower=0  CapacitivePower=3000e6  Pabc=[10e3 9e3 11e3]  QLabc=[100 90 110]  QCabc=[100 90 110]  Pabcp=[10e3 9e3 11e3]  QLabcp=[100 90 110]  QCabcp=[100 90 110]  Measurements=None  LoadType=constant Z
  MTL 4000 MW : powerlib/Elements/Three-Phase Parallel RLC Load  LConnTagsString=A|B|C  Configuration=Y (grounded)  NominalVoltage=(25000)*0.977579  Vabc=[1e3 1e3 1e3]  Vabcp=[1e3 1e3 1e3]  NominalFrequency=60  UnbalancedPower=off  ActivePower=4000000000  InductivePower=0  CapacitivePower=0  Pabc=[10e3 9e3 11e3]  QLabc=[100 90 110]  QCabc=[100 90 110]  Pabcp=[10e3 9e3 11e3]  QLabcp=[100 90 110]  QCabcp=[100 90 110]  Measurements=None  LoadType=constant PQ
  MTL 4000 MW1 : powerlib/Elements/Three-Phase Parallel RLC Load  LConnTagsString=A|B|C  Configuration=Y (grounded)  NominalVoltage=25e3  Vabc=[1e3 1e3 1e3]  Vabcp=[1e3 1e3 1e3]  NominalFrequency=60  UnbalancedPower=off  ActivePower=4000000000  InductivePower=0  CapacitivePower=0  Pabc=[10e3 9e3 11e3]  QLabc=[100 90 110]  QCabc=[100 90 110]  Pabcp=[10e3 9e3 11e3]  QLabcp=[100 90 110]  QCabcp=[100 90 110]  Measurements=None  LoadType=constant Z
  Terminator_1 : Terminator
  Terminator_2 : Terminator
  Tm : Constant  Value=0.80434
  A : PMIOPort  Side=Left
  B : PMIOPort  Port=2  Side=Left
  C : PMIOPort  Port=3  Side=Left
  wires:
  Tm/1 -> ASM 575V 5000MVA Pm=4000 MW/1
  3500 MW/1 -> Terminator_1/1
  ASM 575V 5000MVA Pm=4000 MW/1 -> Terminator_2/1
  connections:
  A/RConn1 -- 22 000 MVA 735 kV/230 kV/LConn1
  B/RConn1 -- 22 000 MVA 735 kV/230 kV/LConn2
  C/RConn1 -- 22 000 MVA 735 kV/230 kV/LConn3
  230 kV/25 kV 18 000 MVA/LConn1 -- Load Flow Bus/LConn1 -- 22 000 MVA 735 kV/230 kV/RConn1 -- MTL 3000 Mvar/LConn1
  230 kV/25 kV 18 000 MVA/LConn2 -- 22 000 MVA 735 kV/230 kV/RConn2 -- MTL 3000 Mvar/LConn2
  230 kV/25 kV 18 000 MVA/LConn3 -- 22 000 MVA 735 kV/230 kV/RConn3 -- MTL 3000 Mvar/LConn3
  MTL 4000 MW1/LConn1 -- Load Flow Bus1/LConn1 -- MTL 4000 MW/LConn1 -- 230 kV/25 kV 18 000 MVA/RConn1 -- 3500 MW/LConn1 -- ASM 575V 5000MVA Pm=4000 MW/LConn1 -- 1.2  Mvar/LConn1
  MTL 4000 MW1/LConn2 -- MTL 4000 MW/LConn2 -- 230 kV/25 kV 18 000 MVA/RConn2 -- 3500 MW/LConn2 -- ASM 575V 5000MVA Pm=4000 MW/LConn2 -- 1.2  Mvar/LConn2
  230 kV/25 kV 18 000 MVA/RConn3 -- ASM 575V 5000MVA Pm=4000 MW/LConn3 -- 1.2  Mvar/LConn3 -- MTL 4000 MW1/LConn3 -- MTL 4000 MW/LConn3 -- 3500 MW/LConn3

== system GFo_29bus/Model Initialization ==
